simulink model "SeyyedAliSadat_DSTATCOM_FACTS_COURSE"  (R2022b)
settings: Solver=FixedStepDiscrete  StartTime=0.0  StopTime=3  FixedStep=Ts  RelTol=1e-3
InitFcn:
  |  Ts=5e-6;
undefined symbols (not defined in the file): D11, Delta, DiscIntNeverNeededParam
libraries: spsSeriesRLCBranchLib x9, spsGroundLib x6, spsThreePhaseVIMeasurementLib x4, spsSecondOrderFilterLib x4, slpidlib x4, spsLinearTransformerLib x3, spsVoltageMeasurementLib x3, spsThreePhaseParallelRLCLoadLib x2, spsUniversalBridgeLib x2, spsabctodq0Lib x2, spsPLL3phLib x2, spsPWMGenerator2LevelLib x2
(part 1 of 2)
Description:
  | Copyright 2008-2014 The MathWorks, Inc.
settings Model: Creator=MathWorks  LastModifiedBy=ali
settings SolverCC: AlgebraicLoopSolver=TrustRegion
settings DataIOCC: SaveFinalState=on  SaveFormat=Structure  SignalLoggingSaveFormat=ModelDataLogs  SaveOutput=off  SaveTime=off  ReturnWorkspaceOutputs=off  SignalLoggingName=sigsOut
settings OptimizationCC: BlockReduction=off  BooleanDataType=off  ExpressionDepthLimit=2147483647  InitFltsAndDblsToZero=on  LifeSpan=inf
settings DebuggingCC: SaveWithParameterizedLinksMsg=none  UnderspecifiedInitializationDetection=Classic  MergeDetectMultiDrivingBlocksExec=none  SignalResolutionControl=TryResolveAllWithWarning  MultiTaskDSMMsg=warning  MultiTaskCondExecSysMsg=none  FcnCallInpInsideContextMsg=warning  UnconnectedInputMsg=warning  UnconnectedOutputMsg=warning  UnconnectedLineMsg=warning  StateNameClashWarn=warning  SFUnexpectedBacktrackingDiag=warning  SFNoUnconditionalDefaultTransitionDiag=warning  SFExecutionAtInitializationDiag=none  SFMachineParentedDataDiag=warning  ArithmeticOperatorsInVariantConditions=warning
settings HardwareCC: ProdBitPerPointer=32  ProdBitPerSizeT=32  ProdBitPerPtrDiffT=32  ProdLargestAtomicFloat=None  ProdIntDivRoundTo=Undefined  ProdEndianess=Unspecified  ProdWordSize=32  ProdHWDeviceType=32-bit Generic  TargetUnknown=on
settings ModelReferenceCC: PropagateSignalLabelsOutOfModel=off
settings SFSimCC: SimUseLocalCustomCode=off  CustomCodeUndefinedFunction=UseInterfaceOnly
settings RTWCC: RTWUseLocalCustomCode=off
settings CodeAppCC: StateflowObjectComments=on
settings GRTTargetCC: TargetFcnLib=ansi_tfl_tmw.mat  TargetLangStandard=C89/C90 (ANSI)  CombineOutputUpdateFcns=off  GRTInterface=on
settings ConfigComp: CovMetricSettings=dw  CovSaveCumulativeToWorkspaceVar=on  CovSaveSingleToWorkspaceVar=on  CovExternalEMLEnable=off  CovSFcnEnable=off
settings SimscapeCC: SimscapeNormalizeSystem=off

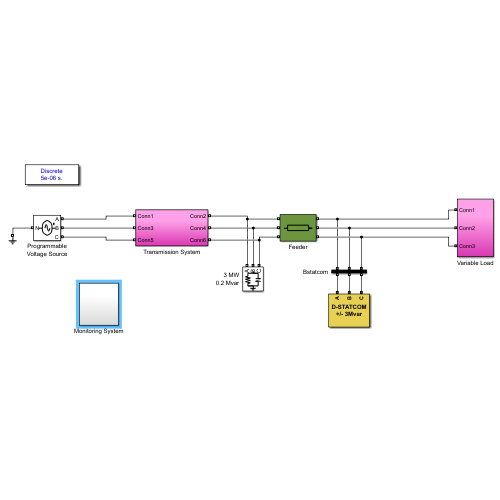
[thumbnail: Simulink's stored preview of the top-level diagram]
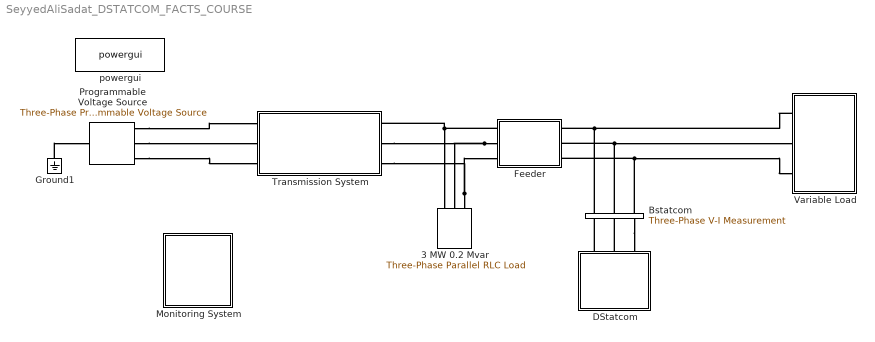
== system SeyyedAliSadat_DSTATCOM_FACTS_COURSE ==
  3 MW 0.2 Mvar : spsThreePhaseParallelRLCLoadLib/Three-Phase Parallel RLC Load  LConnTagsString=A|B|C  Configuration=Y (grounded)  NominalVoltage=33e3  Vabc=[1e3 1e3 1e3]  Vabcp=[1e3 1e3 1e3]  NominalFrequency=60  UnbalancedPower=off  ActivePower=3e6  InductivePower=0  CapacitivePower=0.2e6  Pabc=[10e3 9e3 11e3]  QLabc=[100 90 110]  QCabc=[100 90 110]  Pabcp=[10e3 9e3 11e3]  QLabcp=[100 90 110]  QCabcp=[100 90 110]  Measurements=None  LoadType=constant Z
  Bstatcom : spsThreePhaseVIMeasurementLib/Three-Phase V-I Measurement  VoltageMeasurement=phase-to-ground  SetLabelV=on  LabelV=Vabc_Bstatcom  Vpu=on  VpuLL=off  CurrentMeasurement=yes  SetLabelI=on  LabelI=Iabc_Bstatcom  Ipu=on  Pbase=3e6  Vbase=33e3  OutputType=Magnitude  PhasorSimulation=off  PSBequivalent=0
  DStatcom : Subsystem
      mask Display: disp('D-STATCOM\n+/- 3Mvar')
  Feeder : Subsystem
      mask Display: plot(0,0,100,100,[20,20,80,80,90,80,80,20,20,10],[50,40,40,50,50,50,61,61,50,50])
  Ground1 : spsGroundLib/Ground  LConnTagsString=a
  Monitoring System : Subsystem
  Programmable Voltage Source : spsThreePhaseProgrammableVoltageSourceLib/Three-Phase Programmable Voltage Source  PositiveSequence=[1.077*33e3 19 60]  VariationEntity=None  VariationType=Table of time-amplitude pairs  VariationTypeAlt=Step  VariationStep=0.5  VariationRate=10  VariationMagnitude=0.3  VariationFrequency=2  VariationTiming=[1 2]  VariationPhaseA=off  Amplitudes=[1 1.06 0.94 1.0]  TimeValues="[0 0.4  0.6   0.8 ]"  HarmonicGeneration=off  HarmonicA=[3 0.2 -25 0]  HarmonicB=[2 0.15 35 2]  Timing="[0.05  3]"  BusType=swing  Pref=0  Qref=0  Qmin=-inf  Qmax=inf
  Transmission System : Subsystem
  Variable Load : Subsystem
  powergui : spspowerguiLib/powergui  Priority=2  SimulationMode=Discrete  SampleTime=Ts  frequency=60  Iterations=50  frequencyindice=60  Pbase=100e6  ErrMax=1e-4  UnitsV=kV  UnitsW=MW  buscounter=0  FunctionMessages=off  echomessages=off  EnableUseOfTLC=off  CurrentSourceSwitches=off  DisableSnubberDevices=off  DisableRonSwitches=off  DisableVfSwitches=off  DisplayEquations=off  AutomaticDiscreteSolvers=off  SolverType=Tustin  Interpol=off  ExternalGateDelay=off  methode=off  Ts=0  x0status=blocks  SPID=off  SwTol=0  HookPort=off  NonlinearTolerance=1e-4  nMaxIteration=100  ContinueOnMaxIteration=off  RestoreLinks=warning  ResistiveCurrentMeasurement=off  Frange=[0:2:500]  Ylog=off  Xlog=on  ShowGrid=off  save=off  variable=ZData  structure=Sig1  ZoomFFT=on  StartTime=0.26  cycles=2  DisplayStyle=1  fundamental=60  FreqAxis=off  MaxFrequency=5000  frequencyindicesteady=1  RmsSteady=1  display=off
  connections:
  Bstatcom/LConn1 -- Variable Load/LConn1 -- Feeder/RConn1
  Bstatcom/LConn3 -- Feeder/RConn3 -- Variable Load/LConn3
  Ground1/LConn1 -- Programmable Voltage Source/LConn1
  Feeder/LConn1 -- Transmission System/RConn1 -- 3 MW 0.2 Mvar/LConn1
  Feeder/LConn2 -- Transmission System/RConn2 -- 3 MW 0.2 Mvar/LConn2
  Bstatcom/RConn3 -- DStatcom/RConn3
  DStatcom/RConn1 -- Bstatcom/RConn1
  DStatcom/RConn2 -- Bstatcom/RConn2
  3 MW 0.2 Mvar/LConn3 -- Feeder/LConn3 -- Transmission System/RConn3
  Programmable Voltage Source/RConn1 -- Transmission System/LConn1
  Programmable Voltage Source/RConn2 -- Transmission System/LConn2
  Programmable Voltage Source/RConn3 -- Transmission System/LConn3
  Bstatcom/LConn2 -- Feeder/RConn2 -- Variable Load/LConn2

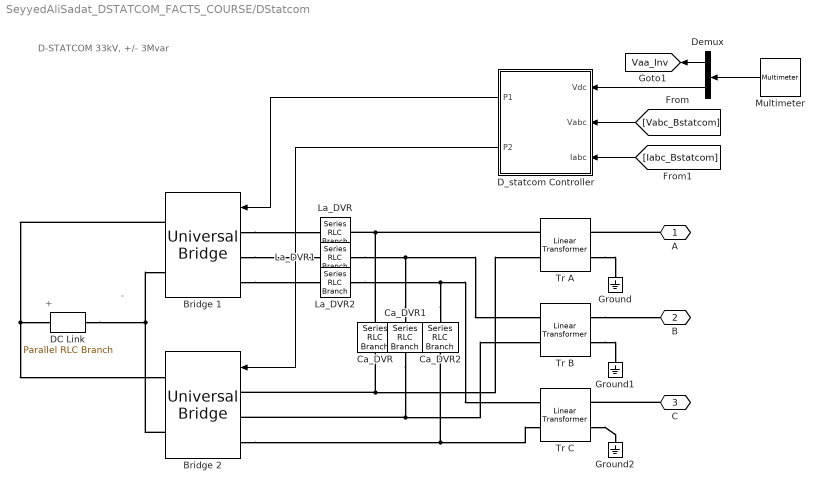
== system SeyyedAliSadat_DSTATCOM_FACTS_COURSE/DStatcom ==
  note: +
  note: -
  note: D-STATCOM
      | 33kV, +/- 3Mvar
  "Bridge 1 " : spsUniversalBridgeLib/Universal Bridge  Arms=3  SnubberResistance=1e5  SnubberCapacitance=inf  Device=IGBT / Diodes  Ron=1e-3  Lon=0  ForwardVoltages="[  2  0.8  ]"  ForwardVoltage=.8  GTOparameters=[ 10e-6 , 20e-6 ]  IGBTparameters=[ 0 0]  Measurements=Device voltages  Measurements_2=None  converterType=Rectifier
      settings: AttributesFormatString=\n
  Bridge 2 : spsUniversalBridgeLib/Universal Bridge  Arms=3  SnubberResistance=1e5  SnubberCapacitance=inf  Device=IGBT / Diodes  Ron=1e-3  Lon=0  ForwardVoltages="[  2  0.8  ]"  ForwardVoltage=.8  GTOparameters=[ 10e-6 , 20e-6 ]  IGBTparameters=[ 0 0]  Measurements=Device voltages  Measurements_2=None  converterType=Rectifier
      settings: AttributesFormatString=\n
  Ca_DVR : spsSeriesRLCBranchLib/Series RLC Branch  LConnTagsString=__new0  RConnTagsString=__new0  BranchType=RC  Resistance=100e-6*(2*pi*60)/40  Inductance=1.0  SetiL0=off  InitialCurrent=0  Capacitance=100e-6  Setx0=off  InitialVoltage=0  Measurements=None
  Ca_DVR1 : spsSeriesRLCBranchLib/Series RLC Branch  LConnTagsString=__new0  RConnTagsString=__new0  BranchType=RC  Resistance=100e-6*(2*pi*60)/40  Inductance=1.0  SetiL0=off  InitialCurrent=0  Capacitance=100e-6  Setx0=off  InitialVoltage=0  Measurements=None
  Ca_DVR2 : spsSeriesRLCBranchLib/Series RLC Branch  LConnTagsString=__new0  RConnTagsString=__new0  BranchType=RC  Resistance=100e-6*(2*pi*60)/40  Inductance=1.0  SetiL0=off  InitialCurrent=0  Capacitance=100e-6  Setx0=off  InitialVoltage=0  Measurements=None
  DC Link : spsParallelRLCBranchLib/Parallel RLC Branch  LConnTagsString=a  RConnTagsString=__new0  BranchType=C  Resistance=1.0  Inductance=1.0  SetiL0=off  InitialCurrent=0  Capacitance=5000e-6  Setx0=off  InitialVoltage=0  Measurements=Branch voltage
  D_statcom Controller : Subsystem  mask(D-STATCOM Controller){ModeOper=Voltage regulation, Vac_Ref=1.0, Qref=0, Vdc_Ref=2400, Par_VacReg=[0.55 2500], Par_VdcReg=[0.001 0.15], Par_IReg=[0.8 200 0], Ts=Ts}
      mask prompts: ModeOper "Mode of operation:"; Vac_Ref "AC voltage setpoint Vref (pu):"; Qref "Manual mode: Qref (Reactive power in pu):"; Vdc_Ref "DC Voltage setpoint (Volts)"; Par_VacReg "Vac Regulator Gains: [ Kp  Ki ]"; Par_VdcReg "Vdc Regulator Gains: [ Kp  Ki ]"; Par_IReg "Current Regulators Gain: [ Kp Ki Kd ]"; Ts "Sample time (s)"
      mask init:
      | Kp_I=Par_IReg(1);
      | Ki_I=Par_IReg(2);
      | Kd_I=Par_IReg(3);
      | Kp_Vdc=Par_VdcReg(1);
      | Ki_Vdc=Par_VdcReg(2);
      | Kp_Vac=Par_VacReg(1);
      | Ki_Vac=Par_VacReg(2);
      mask TypeOptions ModeOper: Voltage regulation | Q regulation
  Demux : Demux  Outputs=[2 1 ]
      settings: DisplayOption=none
  Ground : spsGroundLib/Ground  LConnTagsString=a
  Ground1 : spsGroundLib/Ground  LConnTagsString=a
  Ground2 : spsGroundLib/Ground  LConnTagsString=a
  La_DVR : spsSeriesRLCBranchLib/Series RLC Branch  LConnTagsString=__new0  RConnTagsString=__new0  BranchType=L  Resistance=1.0  Inductance=800e-6  SetiL0=off  InitialCurrent=0  Capacitance=1.0  Setx0=off  InitialVoltage=0  Measurements=None
  La_DVR1 : spsSeriesRLCBranchLib/Series RLC Branch  LConnTagsString=__new0  RConnTagsString=__new0  BranchType=L  Resistance=1.0  Inductance=800e-6  SetiL0=off  InitialCurrent=0  Capacitance=1.0  Setx0=off  InitialVoltage=0  Measurements=None
  La_DVR2 : spsSeriesRLCBranchLib/Series RLC Branch  LConnTagsString=__new0  RConnTagsString=__new0  BranchType=L  Resistance=1.0  Inductance=800e-6  SetiL0=off  InitialCurrent=0  Capacitance=1.0  Setx0=off  InitialVoltage=0  Measurements=None
  Multimeter : spsMultimeterLib/Multimeter  Tag=PoWeRsYsTeMmEaSuReMeNt  L=13  sel=[3 9 1]  yselected={}  Gain=[1 1 1]  OutputType=Magnitude  PlotAtSimulationStop=off  PhasorSimulation=off
      settings: AttributesFormatString=\n
  Tr A : spsLinearTransformerLib/Linear Transformer  UNITS=pu  NominalPower=[3e6/3 60]  winding1=[1250 0.03/30 0.03]  winding2=[33e3/sqrt(3) 0.03/30 0.03]  ThreeWindings=off  winding3=[60e3 0.005 0.02]  RmLm=[200 200]  Measurements=None  DataType=off
  Tr B : spsLinearTransformerLib/Linear Transformer  UNITS=pu  NominalPower=[3e6/3 60]  winding1=[1250 0.03/30 0.03]  winding2=[33e3/sqrt(3) 0.03/30 0.03]  ThreeWindings=off  winding3=[60e3 0.005 0.02]  RmLm=[200 200]  Measurements=None  DataType=off
  Tr C : spsLinearTransformerLib/Linear Transformer  UNITS=pu  NominalPower=[3e6/3 60]  winding1=[1250 0.03/30 0.03]  winding2=[33e3/sqrt(3) 0.03/30 0.03]  ThreeWindings=off  winding3=[60e3 0.005 0.02]  RmLm=[200 200]  Measurements=None  DataType=off
  A : PMIOPort  Side=Right
  B : PMIOPort  Port=2  Side=Right
  C : PMIOPort  Port=3  Side=Right
  tag scope: Vaa_Inv=global
  wires:
  Multimeter/1 -> Demux/1
  Demux/2 -> D_statcom Controller/1(Vdc)
  Demux/1 -> [Vaa_Inv]
  [Vabc_Bstatcom] -> D_statcom Controller/2(Vabc)
  [Iabc_Bstatcom] -> D_statcom Controller/3(Iabc)
  D_statcom Controller/1(P1) -> "Bridge 1 "/1
  D_statcom Controller/2(P2) -> Bridge 2/1
  connections:
  "Bridge 1 "/LConn1 -- La_DVR/LConn1
  "Bridge 1 "/LConn2 -- La_DVR1/LConn1
  "Bridge 1 "/LConn3 -- La_DVR2/LConn1
  Bridge 2/LConn2 -- Tr B/LConn2 -- Ca_DVR1/LConn1
  Bridge 2/LConn3 -- Tr C/LConn2 -- Ca_DVR2/LConn1
  Ca_DVR1/RConn1 -- La_DVR1/RConn1 -- Tr B/LConn1
  Ca_DVR2/RConn1 -- La_DVR2/RConn1 -- Tr C/LConn1
  Tr A/LConn1 -- La_DVR/RConn1 -- Ca_DVR/RConn1
  Tr C/RConn2 -- Ground2/LConn1
  Tr B/RConn2 -- Ground1/LConn1
  Tr A/RConn2 -- Ground/LConn1
  A/RConn1 -- Tr A/RConn1
  Tr B/RConn1 -- B/RConn1
  C/RConn1 -- Tr C/RConn1
  "Bridge 1 "/RConn1 -- Bridge 2/RConn1 -- DC Link/LConn1
  Bridge 2/RConn2 -- "Bridge 1 "/RConn2 -- DC Link/RConn1
  Bridge 2/LConn1 -- Tr A/LConn2 -- Ca_DVR/LConn1

== system SeyyedAliSadat_DSTATCOM_FACTS_COURSE/Feeder ==
  Three-Phase Mutual Inductance Z1-Z0 : spsThreePhaseMutualInductanceZ1Z0Lib/Three-Phase Mutual Inductance Z1-Z0  LConnTagsString=a|b|c  RConnTagsString=A|B|C  PositiveSequence="[0.1153  1.048e-3]*2"  ZeroSequence="[0.3963  2.730e-3]*2"
      settings: AttributesFormatString=\n
      settings: LibrarySourceBlock=|
      | sps_lib/Power Grid Elements/Three-Phase
      | Mutual Inductance
      | Z1-Z0
  A : PMIOPort  Side=Left
  B : PMIOPort  Port=2  Side=Left
  "C " : PMIOPort  Port=3  Side=Left
  a : PMIOPort  Port=4  Side=Right
  b : PMIOPort  Port=5  Side=Right
  c : PMIOPort  Port=6  Side=Right
  connections:
  Three-Phase Mutual Inductance Z1-Z0/RConn3 -- c/RConn1
  Three-Phase Mutual Inductance Z1-Z0/RConn2 -- b/RConn1
  Three-Phase Mutual Inductance Z1-Z0/RConn1 -- a/RConn1
  "C "/RConn1 -- Three-Phase Mutual Inductance Z1-Z0/LConn3
  B/RConn1 -- Three-Phase Mutual Inductance Z1-Z0/LConn2
  A/RConn1 -- Three-Phase Mutual Inductance Z1-Z0/LConn1

== system SeyyedAliSadat_DSTATCOM_FACTS_COURSE/Monitoring System ==
  Data Acquisition : Subsystem
  Demux : Demux  Outputs=2
  Scope1 : Scope  NumInputPorts=2
  Scope2 : Scope  NumInputPorts=4
  Scope3 : Scope  NumInputPorts=3
  Scope4 : Scope  NumInputPorts=2
  Selector : Selector  InputPortWidth=2  IndexOptions=Index vector (dialog)  Indices=2  OutputSizes=1
  wires:
  Data Acquisition/3(Iq_Iqref) -> Scope2/1  "Iq,Iqref (pu)"
  Data Acquisition/2(Va_Inv) -> Scope1/2  "Va Inv (V)"
  Data Acquisition/5(Vdc) -> Scope2/3  "Vdc (V)"
  Data Acquisition/1(VaIa) -> Selector/1, Scope1/1  "Va,Ia (pu)"
  Data Acquisition/4(PQ) -> Scope2/2  "P,Q (MVA)"
  Data Acquisition/6(m) -> Scope2/4
  Selector/1 -> Scope3/3  "Ia STAT (pu)"
  Data Acquisition/7(PQ_B3) -> Scope3/1  "PQ_B3 (MW Mvar)"
  Data Acquisition/8(VmagB1B3) -> Demux/1, Scope3/2  "V_B1 V_B3 (pu)"
  Demux/1 -> Scope4/1
  Demux/2 -> Scope4/2

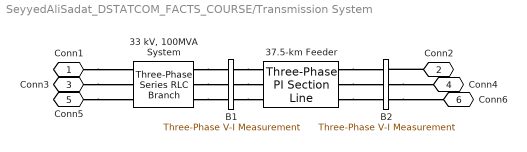
== system SeyyedAliSadat_DSTATCOM_FACTS_COURSE/Transmission System ==
  "33 kV, 100MVA System" : spsThreePhaseSeriesRLCBranchLib/Three-Phase Series RLC Branch  LConnTagsString=A|B|C  RConnTagsString=A|B|C  BranchType=RL  Resistance=33e3^2/100e6/10  Inductance=33e3^2/100e6/(2*pi*60)  Capacitance=1.0  Measurements=None
  37.5-km Feeder : spsThreePhasePISectionLineLib/Three-Phase PI Section Line  LConnTagsString=a|b|c  RConnTagsString=A|B|C  Length=37.5  Frequency=60  Resistances=[0.1153 0.3963]  Inductances=[1.048e-3 2.730e-3]  Capacitances=[11.33e-9 5.338e-9]
  B1 : spsThreePhaseVIMeasurementLib/Three-Phase V-I Measurement  VoltageMeasurement=phase-to-ground  SetLabelV=on  LabelV=Vabc_B1  Vpu=on  VpuLL=off  CurrentMeasurement=no  SetLabelI=off  LabelI=A1  Ipu=off  Pbase=100e6  Vbase=33e3  OutputType=Magnitude  PhasorSimulation=off  PSBequivalent=0
  B2 : spsThreePhaseVIMeasurementLib/Three-Phase V-I Measurement  VoltageMeasurement=phase-to-ground  SetLabelV=on  LabelV=Vabc_B2  Vpu=on  VpuLL=off  CurrentMeasurement=no  SetLabelI=off  LabelI=Iabc_B2  Ipu=off  Pbase=3e6  Vbase=33e3  OutputType=Magnitude  PhasorSimulation=off  PSBequivalent=0
  Conn1 : PMIOPort  Side=Left
  Conn2 : PMIOPort  Port=2  Side=Right
  Conn3 : PMIOPort  Port=3  Side=Left
  Conn4 : PMIOPort  Port=4  Side=Right
  Conn5 : PMIOPort  Port=5  Side=Left
  Conn6 : PMIOPort  Port=6  Side=Right
  connections:
  B1/RConn2 -- 37.5-km Feeder/LConn2
  B2/RConn3 -- Conn6/RConn1
  Conn1/RConn1 -- "33 kV, 100MVA System"/LConn1
  "33 kV, 100MVA System"/RConn3 -- B1/LConn3
  B1/RConn1 -- 37.5-km Feeder/LConn1
  B1/RConn3 -- 37.5-km Feeder/LConn3
  "33 kV, 100MVA System"/RConn2 -- B1/LConn2
  Conn5/RConn1 -- "33 kV, 100MVA System"/LConn3
  37.5-km Feeder/RConn3 -- B2/LConn3
  "33 kV, 100MVA System"/RConn1 -- B1/LConn1
  Conn3/RConn1 -- "33 kV, 100MVA System"/LConn2
  37.5-km Feeder/RConn1 -- B2/LConn1
  37.5-km Feeder/RConn2 -- B2/LConn2
  B2/RConn2 -- Conn4/RConn1
  Conn2/RConn1 -- B2/RConn1

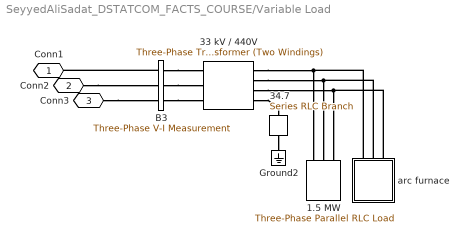
== system SeyyedAliSadat_DSTATCOM_FACTS_COURSE/Variable Load ==
  1.5 MW : spsThreePhaseParallelRLCLoadLib/Three-Phase Parallel RLC Load  LConnTagsString=A|B|C  Configuration=Y (floating)  NominalVoltage=440  Vabc=[1e3 1e3 1e3]  Vabcp=[1e3 1e3 1e3]  NominalFrequency=60  UnbalancedPower=off  ActivePower=1.5e6  InductivePower=0  CapacitivePower=0  Pabc=[10e3 9e3 11e3]  QLabc=[100 90 110]  QCabc=[100 90 110]  Pabcp=[10e3 9e3 11e3]  QLabcp=[100 90 110]  QCabcp=[100 90 110]  Measurements=None  LoadType=constant Z
  33 kV / 440V : spsThreePhaseTransformerTwoWindingsLib/Three-Phase Transformer (Two Windings)  Winding1Connection=Delta (D11)  Winding2Connection=Yn  CoreType=Three single-phase transformers  SetSaturation=off  Hysteresis=off  DataFile='basic_model'  SetInitialFlux=off  Measurements=None  UNITS=pu  NominalPower=[6e6 60]  Winding1=[33e3 , 0.05/30/2 , 0.05]  Winding2=[440 , 0.05/30/2 , 0]  Rm=500  Lm=500  L0=0.5  Saturation="[ 0,0  ;  0.005,1.2  ;  1.0,1.4 ]"  InitialFluxes=[ 0.8 , -0.8 , 0.7 ]  BreakLoop=off  DiscreteSolver=Trapezoidal iterative  DataType=off  TransfoNumber=1
  34.7 : spsSeriesRLCBranchLib/Series RLC Branch  LConnTagsString=__new0  RConnTagsString=__new0  BranchType=R  Resistance=34.7  Inductance=1.0  SetiL0=off  InitialCurrent=0  Capacitance=1.0  Setx0=off  InitialVoltage=0  Measurements=None
  B3 : spsThreePhaseVIMeasurementLib/Three-Phase V-I Measurement  VoltageMeasurement=phase-to-ground  SetLabelV=on  LabelV=Vabc_B3  Vpu=on  VpuLL=off  CurrentMeasurement=yes  SetLabelI=on  LabelI=Iabc_B3  Ipu=on  Pbase=1e6  Vbase=33e3  OutputType=Magnitude  PhasorSimulation=off  PSBequivalent=0
  Ground2 : spsGroundLib/Ground  LConnTagsString=a
  arc furnace : Subsystem  mask(Variable Load (Constant Current)){Par_Nom=[4043.48 0.85], Par_Mod=[3043.48  5], Par_Time=[0.15 1]*1, Vbase=440, Ts=Ts}
      mask prompts: Par_Nom "Nominal load: [ Current (Arms)    Power factor (0 a 1) ]"; Par_Mod "Modulation: [ Amplitude (Arms)   Frequency (Hz) ]"; Par_Time "Modulation timing : [ Ton  Toff ]"; Vbase "Nominal voltage (Volts rms ph-ph)"; Ts "Sample time:"
      mask init:
      | NomAmp=Par_Nom(1)*sqrt(2);
      | NomPha=-acos(Par_Nom(2));
      | ModFreq=Par_Mod(2);
      | ModAmp=Par_Mod(1)*sqrt(2);
      | Ton=Par_Time(1);
      | Toff=Par_Time(2);
  Conn1 : PMIOPort  Side=Left
  Conn2 : PMIOPort  Port=2  Side=Left
  Conn3 : PMIOPort  Port=3  Side=Left
  connections:
  Conn2/RConn1 -- B3/LConn2
  34.7/RConn1 -- Ground2/LConn1
  33 kV / 440V/RConn4 -- 34.7/LConn1
  B3/RConn1 -- 33 kV / 440V/LConn1
  33 kV / 440V/RConn2 -- arc furnace/LConn2 -- 1.5 MW/LConn2
  33 kV / 440V/RConn3 -- arc furnace/LConn3 -- 1.5 MW/LConn3
  B3/RConn2 -- 33 kV / 440V/LConn2
  B3/RConn3 -- 33 kV / 440V/LConn3
  33 kV / 440V/RConn1 -- arc furnace/LConn1 -- 1.5 MW/LConn1
  B3/LConn1 -- Conn1/RConn1
  Conn3/RConn1 -- B3/LConn3

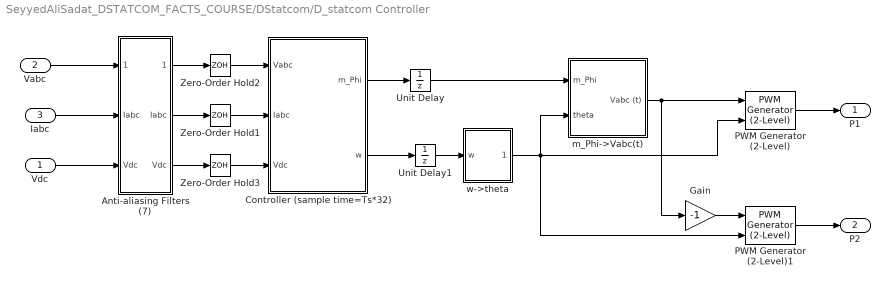
== system SeyyedAliSadat_DSTATCOM_FACTS_COURSE/DStatcom/D_statcom Controller ==
  Vdc : Inport  PortDimensions=1
  Vabc : Inport  Port=2  PortDimensions=3
  Iabc : Inport  Port=3  PortDimensions=3
  Anti-aliasing Filters (7) : Subsystem  mask(Anti-aliasing (2nd order lowpass)){Fc=2000, Ts=Ts}
      mask prompts: Fc "Cut-off frequency (Hz):"; Ts "Sample time:"
  Controller (sample time=Ts*32) : Subsystem
  Gain : Gain  Gain=-1
  PWM Generator (2-Level) : spsPWMGenerator2LevelLib/PWM Generator (2-Level)  ModulatorType=Three-phase bridge (6 pulses)  ModulatorMode=Synchronized  Fc=27*60  Pc=90  nF=28  MinMax="[ -1  1 ]"  SamplingTechnique=Natural  ModulatingSignals=off  m=0.8  Freq=60  Phase=0  Ts=Ts  ShowCarrierOutport=off
  PWM Generator (2-Level)1 : spsPWMGenerator2LevelLib/PWM Generator (2-Level)  ModulatorType=Three-phase bridge (6 pulses)  ModulatorMode=Synchronized  Fc=27*60  Pc=90  nF=28  MinMax="[ -1  1 ]"  SamplingTechnique=Natural  ModulatingSignals=off  m=0.8  Freq=60  Phase=0  Ts=Ts  ShowCarrierOutport=off
  Unit Delay : UnitDelay  SampleTime=Ts*32  HasFrameUpgradeWarning=on
  Unit Delay1 : UnitDelay  SampleTime=Ts*32  HasFrameUpgradeWarning=on
  Zero-Order Hold1 : ZeroOrderHold  SampleTime=Ts*32
  Zero-Order Hold2 : ZeroOrderHold  SampleTime=Ts*32
  Zero-Order Hold3 : ZeroOrderHold  SampleTime=Ts*32
  m_Phi->Vabc(t) : Subsystem
  w->theta : Subsystem
  P1 : Outport
  P2 : Outport  Port=2
  wires:
  Gain/1 -> PWM Generator (2-Level)1/1
  PWM Generator (2-Level)1/1 -> P2/1
  PWM Generator (2-Level)/1 -> P1/1
  Anti-aliasing Filters (7)/1(" Vabc") -> Zero-Order Hold2/1
  Anti-aliasing Filters (7)/2(Iabc) -> Zero-Order Hold1/1
  Anti-aliasing Filters (7)/3(" Vdc") -> Zero-Order Hold3/1
  Vabc/1 -> Anti-aliasing Filters (7)/1(Vabc)
  Iabc/1 -> Anti-aliasing Filters (7)/2("Iabc ")
  Vdc/1 -> Anti-aliasing Filters (7)/3("Vdc ")
  Zero-Order Hold2/1 -> Controller (sample time=Ts*32)/1(Vabc)
  Zero-Order Hold1/1 -> Controller (sample time=Ts*32)/2(Iabc)
  Zero-Order Hold3/1 -> Controller (sample time=Ts*32)/3(Vdc)
  Controller (sample time=Ts*32)/1(m_Phi) -> Unit Delay/1
  Unit Delay/1 -> m_Phi->Vabc(t)/1(m_Phi)
  Controller (sample time=Ts*32)/2(w) -> Unit Delay1/1
  Unit Delay1/1 -> w->theta/1(w)
  m_Phi->Vabc(t)/1(Vabc (t)) -> PWM Generator (2-Level)/1, Gain/1
  w->theta/1(theta) -> PWM Generator (2-Level)/2, m_Phi->Vabc(t)/2(theta), PWM Generator (2-Level)1/2

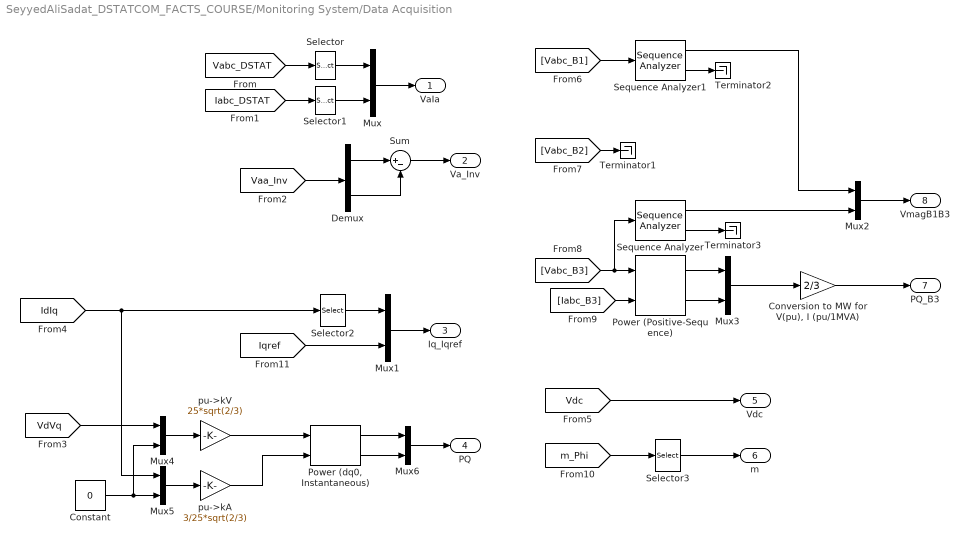
== system SeyyedAliSadat_DSTATCOM_FACTS_COURSE/Monitoring System/Data Acquisition ==
  Constant : Constant  Value=0
  "Conversion to MW for V(pu), I (pu/1MVA)" : Gain  Gain=2/3  SaturateOnIntegerOverflow=on  OutDataTypeStr=Inherit: Same as input  ParamDataTypeStr=Inherit: Same as input
  Demux : Demux  Outputs=2
      settings: DisplayOption=none
  Mux{,1..3,6} (5 alike) : Mux  Inputs=2
  Mux4 : Mux  Inputs=[2,1]
  Mux5 : Mux  Inputs=[2,1]
  Power (Positive-Sequence) : spsPowerPositiveSequenceLib/Power (Positive-Sequence)  Freq=60  Vinit=[1, 0]  Iinit=[0, 0]  Ts=Ts
      settings: LibrarySourceBlock=|
      | sps_lib/Sensors and Measurements/Power
      | (Positive-Sequence)
  "Power (dq0, Instantaneous)" : spsPowerdq0InstantaneousLib/Power (dq0, Instantaneous)
      settings: LibrarySourceBlock=|
      | sps_lib/Sensors and Measurements/Power
      | (dq0, Instantaneous)
  Selector : Selector  InputPortWidth=3  IndexOptions=Index vector (dialog)  Indices=1  OutputSizes=1
  Selector1 : Selector  InputPortWidth=3  IndexOptions=Index vector (dialog)  Indices=1  OutputSizes=1
  Selector2 : Selector  InputPortWidth=2  IndexOptions=Index vector (dialog)  Indices=2  OutputSizes=1
  Selector3 : Selector  InputPortWidth=2  IndexOptions=Index vector (dialog)  Indices=1  OutputSizes=1
  Sequence Analyzer : spsSequenceAnalyzerLib/Sequence Analyzer  Freq=60  n=1  seq=Positive  InInit=[1, 0]  Ts=Ts
      settings: LibrarySourceBlock=sps_lib/Sensors and Measurements/Sequence Analyzer
  Sequence Analyzer1 : spsSequenceAnalyzerLib/Sequence Analyzer  Freq=60  n=1  seq=Positive  InInit=[1, 0]  Ts=Ts
      settings: LibrarySourceBlock=sps_lib/Sensors and Measurements/Sequence Analyzer
  Sum : Sum  Inputs=|+-  SaturateOnIntegerOverflow=on
  Terminator1 : Terminator
  Terminator2 : Terminator
  Terminator3 : Terminator
  pu->kA : Gain  Gain=3/25*sqrt(2/3)  SaturateOnIntegerOverflow=on  OutDataTypeStr=Inherit: Same as input  ParamDataTypeStr=Inherit: Same as input
  pu->kV : Gain  Gain=25*sqrt(2/3)  SaturateOnIntegerOverflow=on  OutDataTypeStr=Inherit: Same as input  ParamDataTypeStr=Inherit: Same as input
  VaIa : Outport
  Va_Inv : Outport  Port=2
  Iq_Iqref : Outport  Port=3
  PQ : Outport  Port=4
  Vdc : Outport  Port=5
  m : Outport  Port=6
  PQ_B3 : Outport  Port=7
  VmagB1B3 : Outport  Port=8
  wires:
  [Vdc] -> Vdc/1
  Selector/1 -> Mux/1
  Selector1/1 -> Mux/2
  Mux/1 -> VaIa/1
  [m_Phi] -> Selector3/1
  [Vabc_DSTAT] -> Selector/1
  [Iabc_DSTAT] -> Selector1/1
  Mux1/1 -> Iq_Iqref/1
  Selector2/1 -> Mux1/1
  [Iqref] -> Mux1/2
  Selector3/1 -> m/1
  [Vaa_Inv] -> Demux/1
  Demux/1 -> Sum/1
  Demux/2 -> Sum/2
  Sum/1 -> Va_Inv/1
  [Vabc_B2] -> Terminator1/1
  [Vabc_B1] -> Sequence Analyzer1/1
  Mux2/1 -> VmagB1B3/1
  "Conversion to MW for V(pu), I (pu/1MVA)"/1 -> PQ_B3/1
  [Iabc_B3] -> Power (Positive-Sequence)/2
  [Vabc_B3] -> Sequence Analyzer/1, Power (Positive-Sequence)/1
  Sequence Analyzer/1 -> Mux2/2
  Power (Positive-Sequence)/1 -> Mux3/1
  Power (Positive-Sequence)/2 -> Mux3/2
  Mux3/1 -> "Conversion to MW for V(pu), I (pu/1MVA)"/1
  Sequence Analyzer/2 -> Terminator3/1
  Sequence Analyzer1/1 -> Mux2/1
  Sequence Analyzer1/2 -> Terminator2/1
  pu->kV/1 -> "Power (dq0, Instantaneous)"/1
  pu->kA/1 -> "Power (dq0, Instantaneous)"/2
  [IdIq] -> Mux5/1, Selector2/1
  [VdVq] -> Mux4/1
  Mux4/1 -> pu->kV/1
  Mux5/1 -> pu->kA/1
  "Power (dq0, Instantaneous)"/1 -> Mux6/1
  "Power (dq0, Instantaneous)"/2 -> Mux6/2
  Mux6/1 -> PQ/1
  Constant/1 -> Mux4/2, Mux5/2

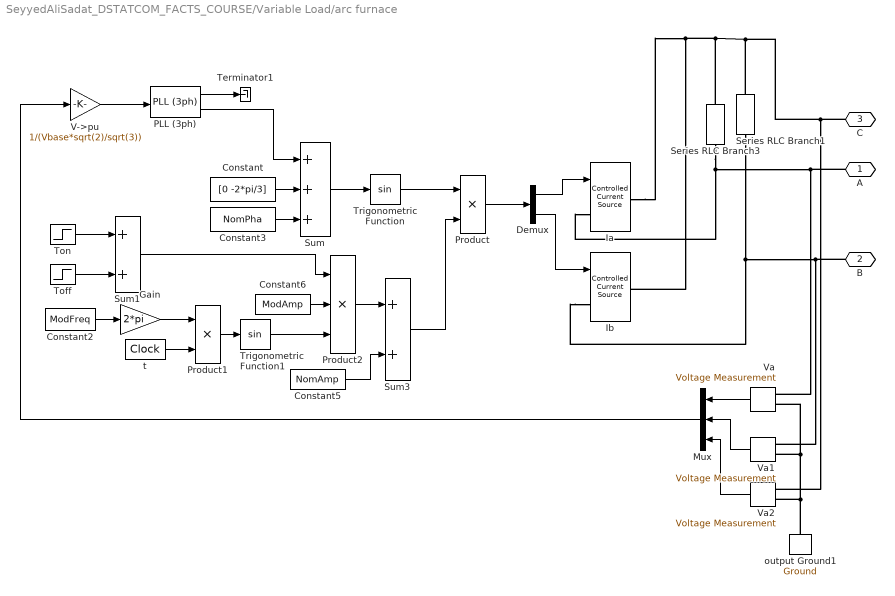
== system SeyyedAliSadat_DSTATCOM_FACTS_COURSE/Variable Load/arc furnace ==
  Constant : Constant  Value=[0 -2*pi/3]
  Constant2 : Constant  Value=ModFreq
  Constant3 : Constant  Value=NomPha
  Constant5 : Constant  Value=NomAmp
  Constant6 : Constant  Value=ModAmp
  Demux : Demux  Outputs=2
      settings: DisplayOption=none
  Gain : Gain  Gain=2*pi  SaturateOnIntegerOverflow=on  OutDataTypeStr=Inherit: Same as input  ParamDataTypeStr=Inherit: Same as input
  Ia : spsControlledCurrentSourceLib/Controlled Current Source  Description=source block  Initialize=on  Source_Type=AC  Amplitude=0  Phase=0  Frequency=0  Measurements=None
      settings: AttributesFormatString=\n
  Ib : spsControlledCurrentSourceLib/Controlled Current Source  Description=source block  Initialize=on  Source_Type=AC  Amplitude=0  Phase=0  Frequency=0  Measurements=None
      settings: AttributesFormatString=\n
  Mux : Mux  Inputs=3
  PLL (3ph) : spsPLL3phLib/PLL (3ph)  Fmin=45  Par_Init=[0, 60]  ParK=[60 1400 0]  TcD=1e-4  MaxRateChangeFreq=12  FilterCutOffFreq=25  Ts=Ts  AGC=off
  Product : Product  InputSameDT=on  SaturateOnIntegerOverflow=on  OutDataTypeStr=Inherit: Same as first input
  Product1 : Product  InputSameDT=on  SaturateOnIntegerOverflow=on  OutDataTypeStr=Inherit: Same as first input
  Product2 : Product  Inputs=3  InputSameDT=on  SaturateOnIntegerOverflow=on  OutDataTypeStr=Inherit: Same as first input
  Series RLC Branch1 : spsSeriesRLCBranchLib/Series RLC Branch  LConnTagsString=__new0  RConnTagsString=__new0  BranchType=R  Resistance=1e6  Inductance=1.0  SetiL0=off  InitialCurrent=0  Capacitance=1.0  Setx0=off  InitialVoltage=0  Measurements=None
  Series RLC Branch3 : spsSeriesRLCBranchLib/Series RLC Branch  LConnTagsString=__new0  RConnTagsString=__new0  BranchType=R  Resistance=1e6  Inductance=1.0  SetiL0=off  InitialCurrent=0  Capacitance=1.0  Setx0=off  InitialVoltage=0  Measurements=None
  Sum : Sum  Inputs=+++  InputSameDT=on  SaturateOnIntegerOverflow=on  OutDataTypeStr=Inherit: Same as first input
  Sum1 : Sum  InputSameDT=on  SaturateOnIntegerOverflow=on  OutDataTypeStr=Inherit: Same as first input
  Sum3 : Sum  InputSameDT=on  SaturateOnIntegerOverflow=on  OutDataTypeStr=Inherit: Same as first input
  Terminator1 : Terminator
  Toff : Step  Time=Toff  After=-1  SampleTime=Ts
  Ton : Step  Time=Ton  SampleTime=Ts
  Trigonometric Function : Trigonometry
  Trigonometric Function1 : Trigonometry
  V->pu : Gain  Gain=1/(Vbase*sqrt(2)/sqrt(3))  SaturateOnIntegerOverflow=on  OutDataTypeStr=Inherit: Same as input  ParamDataTypeStr=Inherit: Same as input
  Va : spsVoltageMeasurementLib/Voltage Measurement  Tag=PoWeRsYsTeMmEaSuReMeNt  PhasorSimulation=off  OutputType=Magnitude  PSBequivalent=0
  Va1 : spsVoltageMeasurementLib/Voltage Measurement  Tag=PoWeRsYsTeMmEaSuReMeNt  PhasorSimulation=off  OutputType=Magnitude  PSBequivalent=0
  Va2 : spsVoltageMeasurementLib/Voltage Measurement  Tag=PoWeRsYsTeMmEaSuReMeNt  PhasorSimulation=off  OutputType=Magnitude  PSBequivalent=0
  output Ground1 : spsGroundLib/Ground  LConnTagsString=a  RConnTagsString=__newr0
  t : DigitalClock  SampleTime=Ts
  A : PMIOPort  Side=Left
  B : PMIOPort  Port=2  Side=Left
  C : PMIOPort  Port=3  Side=Left
  wires:
  Sum1/1 -> Product2/1
  Toff/1 -> Sum1/2
  Ton/1 -> Sum1/1
  Constant6/1 -> Product2/2
  Trigonometric Function1/1 -> Product2/3
  Constant5/1 -> Sum3/2
  Product2/1 -> Sum3/1
  Sum3/1 -> Product/2
  Product1/1 -> Trigonometric Function1/1
  t/1 -> Product1/2
  Gain/1 -> Product1/1
  Constant2/1 -> Gain/1
  Constant3/1 -> Sum/3
  Mux/1 -> V->pu/1
  V->pu/1 -> PLL (3ph)/1
  Product/1 -> Demux/1
  Trigonometric Function/1 -> Product/1
  Sum/1 -> Trigonometric Function/1
  Constant/1 -> Sum/2
  Va2/1 -> Mux/3
  Va1/1 -> Mux/2
  Va/1 -> Mux/1
  Demux/1 -> Ia/1
  Demux/2 -> Ib/1
  PLL (3ph)/2 -> Sum/1
  PLL (3ph)/1 -> Terminator1/1
  connections:
  output Ground1/LConn1 -- Va2/LConn2 -- Va1/LConn2 -- Va/LConn2
  Ib/LConn1 -- Series RLC Branch1/LConn1 -- B/RConn1 -- Va1/LConn1
  Ia/LConn1 -- Series RLC Branch3/LConn1 -- A/RConn1 -- Va/LConn1
  Series RLC Branch1/RConn1 -- Series RLC Branch3/RConn1 -- Ia/RConn1 -- Ib/RConn1 -- C/RConn1 -- Va2/LConn1

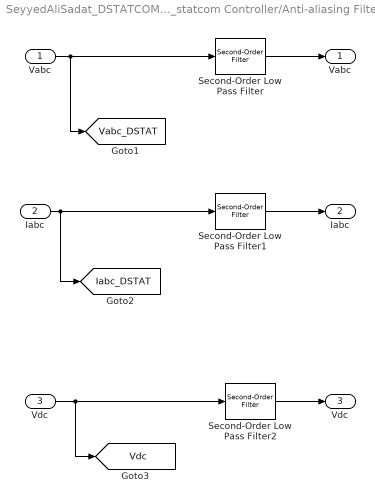
== system SeyyedAliSadat_DSTATCOM_FACTS_COURSE/DStatcom/D_statcom Controller/Anti-aliasing Filters (7) ==
  Vabc : Inport  PortDimensions=3
  "Iabc " : Inport  Port=2  PortDimensions=3
  "Vdc " : Inport  Port=3  PortDimensions=1
  Second-Order Low Pass Filter : spsSecondOrderFilterLib/Second-Order Filter  FilterType=Lowpass  Fo=Fc  Zeta=0.707  Ts=Ts  Initialize=off  Vac_Init="[0,  0,  60]"  Vdc_Init=0  PlotResponse=off  FreqRange=[0, 500, 1]
      settings: AttributesFormatString=f0: %<Fo>
      settings: LibrarySourceBlock=|
      | sps_lib/Control/Filters/Second-Order
      | Filter
  Second-Order Low Pass Filter1 : spsSecondOrderFilterLib/Second-Order Filter  FilterType=Lowpass  Fo=Fc  Zeta=0.707  Ts=Ts  Initialize=off  Vac_Init="[0,  0,  60]"  Vdc_Init=0  PlotResponse=off  FreqRange=[0, 500, 1]
      settings: AttributesFormatString=f0: %<Fo>
      settings: LibrarySourceBlock=|
      | sps_lib/Control/Filters/Second-Order
      | Filter
  Second-Order Low Pass Filter2 : spsSecondOrderFilterLib/Second-Order Filter  FilterType=Lowpass  Fo=Fc  Zeta=0.707  Ts=Ts  Initialize=off  Vac_Init="[0,  0,  60]"  Vdc_Init=0  PlotResponse=off  FreqRange=[0, 500, 1]
      settings: AttributesFormatString=f0: %<Fo>
      settings: LibrarySourceBlock=|
      | sps_lib/Control/Filters/Second-Order
      | Filter
  " Vabc" : Outport
  Iabc : Outport  Port=2
  " Vdc" : Outport  Port=3
  tag scope: Iabc_DSTAT=global, Vabc_DSTAT=global, Vdc=global
  wires:
  Second-Order Low Pass Filter/1 -> " Vabc"/1
  Second-Order Low Pass Filter1/1 -> Iabc/1
  "Iabc "/1 -> [Iabc_DSTAT], Second-Order Low Pass Filter1/1
  Vabc/1 -> [Vabc_DSTAT], Second-Order Low Pass Filter/1
  "Vdc "/1 -> [Vdc], Second-Order Low Pass Filter2/1
  Second-Order Low Pass Filter2/1 -> " Vdc"/1

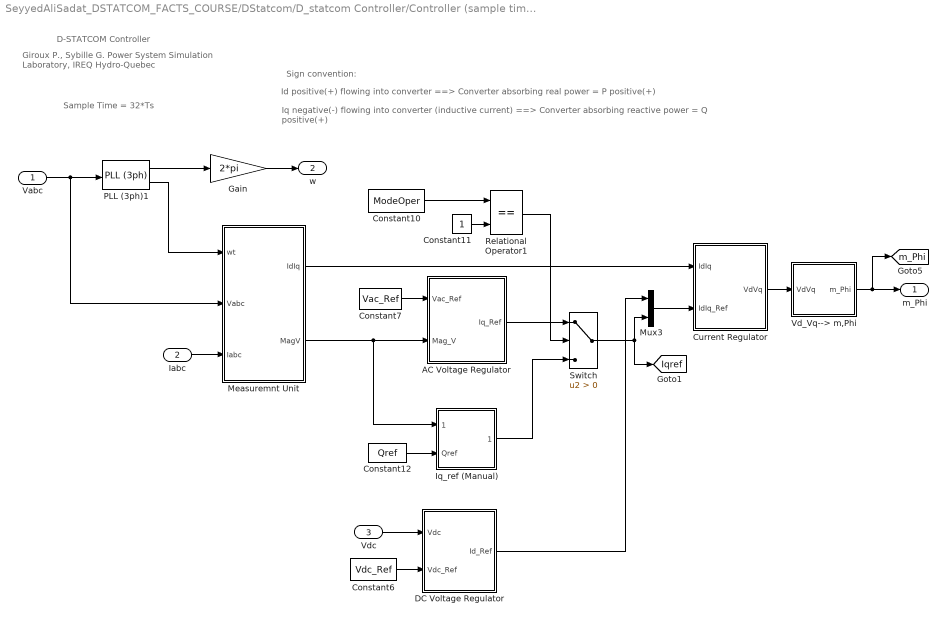
== system SeyyedAliSadat_DSTATCOM_FACTS_COURSE/DStatcom/D_statcom Controller/Controller (sample time=Ts*32) ==
  note: Sample Time = 32*Ts
  note: Id positive(+) flowing into converter ==> Converter absorbing real power = P positive(+)
  note: Sign convention:
  note: Iq negative(-) flowing into converter (inductive current) ==> Converter absorbing reactive power = Q positive(+)
  note: Giroux P., Sybille G.
      | Power System Simulation Laboratory, IREQ
      | Hydro-Quebec
  note: D-STATCOM Controller
  Vabc : Inport  PortDimensions=3
  Iabc : Inport  Port=2  PortDimensions=3
  Vdc : Inport  Port=3  PortDimensions=1
  AC Voltage Regulator : Subsystem  mask(DC Voltage regulator){Kp=Kp_Vac, Ki=Ki_Vac, Ts=32*Ts}
      mask prompts: Kp "Proportional gain (Kp):"; Ki "Integral gain(Ki)"; Ts "Sample time:"
  Constant10 : Constant  Value=ModeOper
  Constant11 : Constant
  Constant12 : Constant  Value=Qref
  Constant6 : Constant  Value=Vdc_Ref
  Constant7 : Constant  Value=Vac_Ref
  Current Regulator : Subsystem  mask(Current Regulators){Kp=Kp_I, Ki=Ki_I, Par_Limits=[1 -1], Init=0, Ts=32*Ts}
      mask prompts: Kp "Proportional gain (Kp):"; Ki "Integral gain (Ki):"; Par_Limits "Output limits: [ Upper   Lower ]"; Init "Output initial value:"; Ts "Sample time:"
      mask help:
      | Sign convention:
      | Id positive(+) flowing into converter ==> Converter absorbing real power = P positive(+)
      | Iq negative(-) flowing into converter (inductive current) ==> Converter absorbing reactive power = Q positive(+)
  DC Voltage Regulator : Subsystem  mask(DC Voltage regulator){Kp=Kp_Vdc, Ki=Ki_Vdc, Ts=32*Ts}
      mask prompts: Kp "Proportional gain (Kp):"; Ki "Integral gain(Ki)"; Ts "Sample time:"
  Gain : Gain  Gain=2*pi
  Iq_ref (Manual) : Subsystem
  Measuremnt Unit : Subsystem
  Mux3 : Mux  Inputs=2
  PLL (3ph)1 : spsPLL3phLib/PLL (3ph)  Fmin=45  Par_Init=[3.7 60]  ParK=[60 1400 0]  TcD=1.6e-4  MaxRateChangeFreq=10  FilterCutOffFreq=25  Ts=32*Ts  AGC=off
  Relational Operator1 : RelationalOperator  Operator===
  Switch : Switch  Criteria=u2 > Threshold
  Vd_Vq--> m,Phi : Subsystem
  m_Phi : Outport
  w : Outport  Port=2
  tag scope: Iqref=global, m_Phi=global
  wires:
  Gain/1 -> w/1
  PLL (3ph)1/1 -> Gain/1
  PLL (3ph)1/2 -> Measuremnt Unit/1(wt)
  Vabc/1 -> Measuremnt Unit/2(Vabc), PLL (3ph)1/1
  Constant6/1 -> DC Voltage Regulator/2(Vdc_Ref)
  Vdc/1 -> DC Voltage Regulator/1(Vdc)
  Constant11/1 -> Relational Operator1/2
  Constant10/1 -> Relational Operator1/1
  Constant12/1 -> Iq_ref (Manual)/2(Qref)
  Iabc/1 -> Measuremnt Unit/3(Iabc)
  Measuremnt Unit/2(MagV) -> AC Voltage Regulator/2(Mag_V), Iq_ref (Manual)/1(MagV)
  Constant7/1 -> AC Voltage Regulator/1(Vac_Ref)
  Measuremnt Unit/1(IdIq) -> Current Regulator/1(IdIq)
  AC Voltage Regulator/1(Iq_Ref) -> Switch/1
  Mux3/1 -> Current Regulator/2(IdIq_Ref)
  Switch/1 -> Mux3/2, [Iqref]
  DC Voltage Regulator/1(Id_Ref) -> Mux3/1
  Iq_ref (Manual)/1(Iqref*) -> Switch/3
  Relational Operator1/1 -> Switch/2
  Current Regulator/1(VdVq) -> Vd_Vq--> m,Phi/1(VdVq)
  Vd_Vq--> m,Phi/1(m_Phi) -> m_Phi/1, [m_Phi]

== system SeyyedAliSadat_DSTATCOM_FACTS_COURSE/DStatcom/D_statcom Controller/m_Phi->Vabc(t) ==
  m_Phi : Inport
  theta : Inport  Port=2
  Constant1 : Constant  Value=[0 -2*pi/3 2*pi/3]
  Demux : Demux  Outputs=2
      settings: DisplayOption=none
  Product2 : Product  InputSameDT=on  SaturateOnIntegerOverflow=on  OutDataTypeStr=Inherit: Same as first input
  Sum4 : Sum  Inputs=+++  InputSameDT=on  SaturateOnIntegerOverflow=on  OutDataTypeStr=Inherit: Same as first input
  Trigonometric Function1 : Trigonometry
  deg. ->rad : Gain  Gain=pi/180  SaturateOnIntegerOverflow=on  OutDataTypeStr=Inherit: Same as input  ParamDataTypeStr=Inherit: Same as input
  Vabc (t) : Outport
  wires:
  Trigonometric Function1/1 -> Product2/2
  Sum4/1 -> Trigonometric Function1/1
  Constant1/1 -> Sum4/2
  Demux/1 -> Product2/1
  Product2/1 -> Vabc (t)/1
  m_Phi/1 -> Demux/1
  deg. ->rad/1 -> Sum4/1
  theta/1 -> Sum4/3
  Demux/2 -> deg. ->rad/1

== system SeyyedAliSadat_DSTATCOM_FACTS_COURSE/DStatcom/D_statcom Controller/w->theta ==
  w : Inport
  Constant4 : Constant  Value=2*pi
  Discrete-Time Integrator : DiscreteIntegrator  SampleTime=Ts  ICPrevOutput=DiscIntNeverNeededParam  ICPrevScaledInput=DiscIntNeverNeededParam
  Math Function : Math  Operator=mod  SignedPower=on
  theta : Outport
  wires:
  Math Function/1 -> theta/1
  w/1 -> Discrete-Time Integrator/1
  Constant4/1 -> Math Function/2
  Discrete-Time Integrator/1 -> Math Function/1

== system SeyyedAliSadat_DSTATCOM_FACTS_COURSE/DStatcom/D_statcom Controller/Controller (sample time=Ts*32)/AC Voltage Regulator ==
  Vac_Ref : Inport
  Mag_V : Inport  Port=2
  Discrete PI Controller : slpidlib/PID Controller  Controller=PI  Form=Parallel  TimeDomain=Discrete-time  UseExternalTs=off  SampleTime=Ts  IntegratorMethod=Forward Euler  FilterMethod=Forward Euler  ControllerParametersSource=internal  P=Kp  I=Ki  UseKiTs=off  D=0  N=100  UseFilter=on  TunerSelectOption=Transfer Function Based (PID Tuner App)  InitialConditionSource=internal  InitialConditionForIntegrator=0  InitialConditionForFilter=0  DifferentiatorICPrevScaledInput=0  ExternalReset=none  TrackingMode=off  Kt=1  LimitOutput=on  SatLimitsSource=internal  UpperSaturationLimit=1  LowerSaturationLimit=-1  LinearizeAsGain=off  AntiWindupMode=clamping  Kb=1  LimitIntegrator=off  UpperIntegratorSaturationLimit=inf  LowerIntegratorSaturationLimit=-inf  POutMin=[]  POutMax=[]  IOutMin=[]  IOutMax=[]  DOutMin=[]  DOutMax=[]  NOutMin=[]  NOutMax=[]  SumOutMin=[]  SumOutMax=[]  SaturationOutMin=[]  SaturationOutMax=[]  PParamMin=[]  PParamMax=[]  IParamMin=[]  IParamMax=[]  DParamMin=[]  DParamMax=[]  NParamMin=[]  NParamMax=[]  KbParamMin=[]  KbParamMax=[]  KtParamMin=[]  KtParamMax=[]  KbOutMin=[]  KbOutMax=[]  KtOutMin=[]  KtOutMax=[]  IntegratorOutMin=[]  IntegratorOutMax=[]  FilterOutMin=[]  FilterOutMax=[]  SumI1OutMin=[]  SumI1OutMax=[]  SumI2OutMin=[]  SumI2OutMax=[]  SumI3OutMin=[]  SumI3OutMax=[]  SumI4OutMin=[]  SumI4OutMax=[]  SumDOutMin=[]  SumDOutMax=[]  DifferentiatorOutMin=[]  DifferentiatorOutMax=[]  FilterDiffOutCoefMin=[]  FilterDiffOutCoefMax=[]  ReciprocalOutMin=[]  ReciprocalOutMax=[]  SumDenOutMin=[]  SumDenOutMax=[]  SumNumOutMin=[]  SumNumOutMax=[]  DivideOutMin=[]  DivideOutMax=[]  UdiffTsProdOutMin=[]  UdiffTsProdOutMax=[]  NTsProdOutMin=[]  NTsProdOutMax=[]  UintegralTsProdOutMin=[]  UintegralTsProdOutMax=[]  UngainTsProdOutMin=[]  UngainTsProdOutMax=[]  ClampingZeroOutDataTypeStr=Inherit: Inherit via back propagation  ClampingZeroOutMin=[]  ClampingZeroOutMax=[]  FilterDenConstantOutDataTypeStr=Inherit: Inherit via back propagation  FilterDenConstantOutMin=[]  FilterDenConstantOutMax=[]  PCopyOutDataTypeStr=Inherit: Inherit via back propagation  PCopyOutMin=[]  PCopyOutMax=[]  NCopyOutDataTypeStr=Inherit: Inherit via back propagation  NCopyOutMin=[]  NCopyOutMax=[]  IntegratorContinuousStateAttributes=''  IntegratorStateMustResolveToSignalObject=off  IntegratorRTWStateStorageClass=Auto  FilterContinuousStateAttributes=''  FilterStateMustResolveToSignalObject=off  FilterRTWStateStorageClass=Auto  ParallelPVariant=InternalParameters  IdealPVariant=Disabled  IVariant=InternalParameters  DVariant=Disabled  IntegratorVariant=Discrete  SatVariant=Enabled  AWVariant=DiscClampingParallel  PCopyVariant=Disabled  TRVariant=Disabled  FdbkBlocksVariant=Forward  IdealPFdbkVariant=Disabled  SatFdbkVariant=Disabled  DerivativeFilterVariant=Disabled  NVariant=Disabled  NCopyVariant=Disabled_SignalSpec  FilterICVariant=Disabled  IntegratorICVariant=InternalICs  ExternalResetVariant=Disabled  TRSumVariant=Passthrough  SumFdbkVariant=Disabled  SumVariant=Sum_PI  TsampFilterVariant=InternalTs  TsampNgainVariant=Passthrough  TsampIntegralVariant=Passthrough  ExternalSaturationOutDataTypeStr=Inherit: Same as second input
      settings: AttributesFormatString=P = %<P>\nI = %<I>
  Sum : Sum  Inputs=|+-  InputSameDT=on  SaturateOnIntegerOverflow=on  OutDataTypeStr=Inherit: Same as first input
  Iq_Ref : Outport  InitialOutput=0
  wires:
  Discrete PI Controller/1 -> Iq_Ref/1
  Sum/1 -> Discrete PI Controller/1
  Mag_V/1 -> Sum/2
  Vac_Ref/1 -> Sum/1

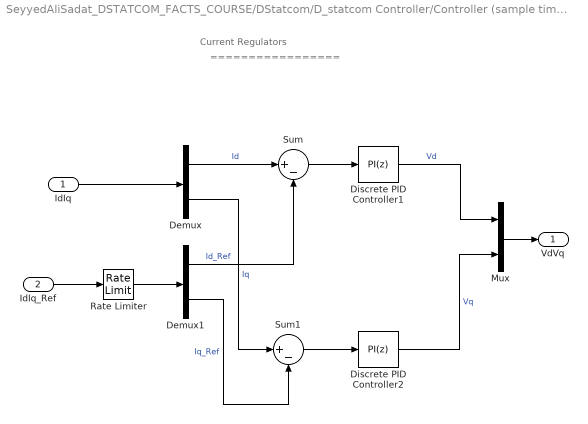
== system SeyyedAliSadat_DSTATCOM_FACTS_COURSE/DStatcom/D_statcom Controller/Controller (sample time=Ts*32)/Current Regulator ==
  note: Current Regulators
  note: =================
  IdIq : Inport  PortDimensions=2
  IdIq_Ref : Inport  Port=2  PortDimensions=2
  Demux : Demux  Outputs=2
      settings: DisplayOption=none
  Demux1 : Demux  Outputs=2
      settings: DisplayOption=none
  Discrete PID Controller1 : slpidlib/PID Controller  Controller=PI  Form=Parallel  TimeDomain=Discrete-time  UseExternalTs=off  SampleTime=Ts  IntegratorMethod=Forward Euler  FilterMethod=Forward Euler  ControllerParametersSource=internal  P=Kp  I=Ki  UseKiTs=off  D=0  N=100  UseFilter=on  TunerSelectOption=Transfer Function Based (PID Tuner App)  InitialConditionSource=internal  InitialConditionForIntegrator=0  InitialConditionForFilter=0  DifferentiatorICPrevScaledInput=0  ExternalReset=none  TrackingMode=off  Kt=1  LimitOutput=on  SatLimitsSource=internal  UpperSaturationLimit=1  LowerSaturationLimit=-1  LinearizeAsGain=off  AntiWindupMode=clamping  Kb=1  LimitIntegrator=off  UpperIntegratorSaturationLimit=inf  LowerIntegratorSaturationLimit=-inf  POutMin=[]  POutMax=[]  IOutMin=[]  IOutMax=[]  DOutMin=[]  DOutMax=[]  NOutMin=[]  NOutMax=[]  SumOutMin=[]  SumOutMax=[]  SaturationOutMin=[]  SaturationOutMax=[]  PParamMin=[]  PParamMax=[]  IParamMin=[]  IParamMax=[]  DParamMin=[]  DParamMax=[]  NParamMin=[]  NParamMax=[]  KbParamMin=[]  KbParamMax=[]  KtParamMin=[]  KtParamMax=[]  KbOutMin=[]  KbOutMax=[]  KtOutMin=[]  KtOutMax=[]  IntegratorOutMin=[]  IntegratorOutMax=[]  FilterOutMin=[]  FilterOutMax=[]  SumI1OutMin=[]  SumI1OutMax=[]  SumI2OutMin=[]  SumI2OutMax=[]  SumI3OutMin=[]  SumI3OutMax=[]  SumI4OutMin=[]  SumI4OutMax=[]  SumDOutMin=[]  SumDOutMax=[]  DifferentiatorOutMin=[]  DifferentiatorOutMax=[]  FilterDiffOutCoefMin=[]  FilterDiffOutCoefMax=[]  ReciprocalOutMin=[]  ReciprocalOutMax=[]  SumDenOutMin=[]  SumDenOutMax=[]  SumNumOutMin=[]  SumNumOutMax=[]  DivideOutMin=[]  DivideOutMax=[]  UdiffTsProdOutMin=[]  UdiffTsProdOutMax=[]  NTsProdOutMin=[]  NTsProdOutMax=[]  UintegralTsProdOutMin=[]  UintegralTsProdOutMax=[]  UngainTsProdOutMin=[]  UngainTsProdOutMax=[]  ClampingZeroOutDataTypeStr=Inherit: Inherit via back propagation  ClampingZeroOutMin=[]  ClampingZeroOutMax=[]  FilterDenConstantOutDataTypeStr=Inherit: Inherit via back propagation  FilterDenConstantOutMin=[]  FilterDenConstantOutMax=[]  PCopyOutDataTypeStr=Inherit: Inherit via back propagation  PCopyOutMin=[]  PCopyOutMax=[]  NCopyOutDataTypeStr=Inherit: Inherit via back propagation  NCopyOutMin=[]  NCopyOutMax=[]  IntegratorContinuousStateAttributes=''  IntegratorStateMustResolveToSignalObject=off  IntegratorRTWStateStorageClass=Auto  FilterContinuousStateAttributes=''  FilterStateMustResolveToSignalObject=off  FilterRTWStateStorageClass=Auto  ParallelPVariant=InternalParameters  IdealPVariant=Disabled  IVariant=InternalParameters  DVariant=Disabled  IntegratorVariant=Discrete  SatVariant=Enabled  AWVariant=DiscClampingParallel  PCopyVariant=Disabled  TRVariant=Disabled  FdbkBlocksVariant=Forward  IdealPFdbkVariant=Disabled  SatFdbkVariant=Disabled  DerivativeFilterVariant=Disabled  NVariant=Disabled  NCopyVariant=Disabled_SignalSpec  FilterICVariant=Disabled  IntegratorICVariant=InternalICs  ExternalResetVariant=Disabled  TRSumVariant=Passthrough  SumFdbkVariant=Disabled  SumVariant=Sum_PI  TsampFilterVariant=InternalTs  TsampNgainVariant=Passthrough  TsampIntegralVariant=Passthrough  ExternalSaturationOutDataTypeStr=Inherit: Same as second input
      settings: AttributesFormatString=P = %<P>\nI = %<I>
  Discrete PID Controller2 : slpidlib/PID Controller  Controller=PI  Form=Parallel  TimeDomain=Discrete-time  UseExternalTs=off  SampleTime=Ts  IntegratorMethod=Forward Euler  FilterMethod=Forward Euler  ControllerParametersSource=internal  P=Kp  I=Ki  UseKiTs=off  D=0  N=100  UseFilter=on  TunerSelectOption=Transfer Function Based (PID Tuner App)  InitialConditionSource=internal  InitialConditionForIntegrator=0  InitialConditionForFilter=0  DifferentiatorICPrevScaledInput=0  ExternalReset=none  TrackingMode=off  Kt=1  LimitOutput=on  SatLimitsSource=internal  UpperSaturationLimit=1  LowerSaturationLimit=-1  LinearizeAsGain=off  AntiWindupMode=clamping  Kb=1  LimitIntegrator=off  UpperIntegratorSaturationLimit=inf  LowerIntegratorSaturationLimit=-inf  POutMin=[]  POutMax=[]  IOutMin=[]  IOutMax=[]  DOutMin=[]  DOutMax=[]  NOutMin=[]  NOutMax=[]  SumOutMin=[]  SumOutMax=[]  SaturationOutMin=[]  SaturationOutMax=[]  PParamMin=[]  PParamMax=[]  IParamMin=[]  IParamMax=[]  DParamMin=[]  DParamMax=[]  NParamMin=[]  NParamMax=[]  KbParamMin=[]  KbParamMax=[]  KtParamMin=[]  KtParamMax=[]  KbOutMin=[]  KbOutMax=[]  KtOutMin=[]  KtOutMax=[]  IntegratorOutMin=[]  IntegratorOutMax=[]  FilterOutMin=[]  FilterOutMax=[]  SumI1OutMin=[]  SumI1OutMax=[]  SumI2OutMin=[]  SumI2OutMax=[]  SumI3OutMin=[]  SumI3OutMax=[]  SumI4OutMin=[]  SumI4OutMax=[]  SumDOutMin=[]  SumDOutMax=[]  DifferentiatorOutMin=[]  DifferentiatorOutMax=[]  FilterDiffOutCoefMin=[]  FilterDiffOutCoefMax=[]  ReciprocalOutMin=[]  ReciprocalOutMax=[]  SumDenOutMin=[]  SumDenOutMax=[]  SumNumOutMin=[]  SumNumOutMax=[]  DivideOutMin=[]  DivideOutMax=[]  UdiffTsProdOutMin=[]  UdiffTsProdOutMax=[]  NTsProdOutMin=[]  NTsProdOutMax=[]  UintegralTsProdOutMin=[]  UintegralTsProdOutMax=[]  UngainTsProdOutMin=[]  UngainTsProdOutMax=[]  ClampingZeroOutDataTypeStr=Inherit: Inherit via back propagation  ClampingZeroOutMin=[]  ClampingZeroOutMax=[]  FilterDenConstantOutDataTypeStr=Inherit: Inherit via back propagation  FilterDenConstantOutMin=[]  FilterDenConstantOutMax=[]  PCopyOutDataTypeStr=Inherit: Inherit via back propagation  PCopyOutMin=[]  PCopyOutMax=[]  NCopyOutDataTypeStr=Inherit: Inherit via back propagation  NCopyOutMin=[]  NCopyOutMax=[]  IntegratorContinuousStateAttributes=''  IntegratorStateMustResolveToSignalObject=off  IntegratorRTWStateStorageClass=Auto  FilterContinuousStateAttributes=''  FilterStateMustResolveToSignalObject=off  FilterRTWStateStorageClass=Auto  ParallelPVariant=InternalParameters  IdealPVariant=Disabled  IVariant=InternalParameters  DVariant=Disabled  IntegratorVariant=Discrete  SatVariant=Enabled  AWVariant=DiscClampingParallel  PCopyVariant=Disabled  TRVariant=Disabled  FdbkBlocksVariant=Forward  IdealPFdbkVariant=Disabled  SatFdbkVariant=Disabled  DerivativeFilterVariant=Disabled  NVariant=Disabled  NCopyVariant=Disabled_SignalSpec  FilterICVariant=Disabled  IntegratorICVariant=InternalICs  ExternalResetVariant=Disabled  TRSumVariant=Passthrough  SumFdbkVariant=Disabled  SumVariant=Sum_PI  TsampFilterVariant=InternalTs  TsampNgainVariant=Passthrough  TsampIntegralVariant=Passthrough  ExternalSaturationOutDataTypeStr=Inherit: Same as second input
      settings: AttributesFormatString=P = %<P>\nI = %<I>
  Mux : Mux  Inputs=2
  Rate Limiter : RateLimiter  RisingSlewLimit=240  FallingSlewLimit=-240  SampleTimeMode=inherited
      settings: AttributesFormatString=Up = %<RisingSlewLimit>\nDown = %<FallingSlewLimit>\nIC = %<InitialCondition>
  Sum : Sum  Inputs=|+-  InputSameDT=on  SaturateOnIntegerOverflow=on  OutDataTypeStr=Inherit: Same as first input
  Sum1 : Sum  Inputs=|+-  InputSameDT=on  SaturateOnIntegerOverflow=on  OutDataTypeStr=Inherit: Same as first input
  VdVq : Outport
  wires:
  Discrete PID Controller2/1 -> Mux/2  "Vq"
  Discrete PID Controller1/1 -> Mux/1  "Vd"
  IdIq/1 -> Demux/1
  Demux/1 -> Sum/1  "Id"
  Demux1/1 -> Sum/2  "Id_Ref"
  Demux/2 -> Sum1/1  "Iq"
  Sum1/1 -> Discrete PID Controller2/1
  Demux1/2 -> Sum1/2  "Iq_Ref"
  Sum/1 -> Discrete PID Controller1/1
  Mux/1 -> VdVq/1
  IdIq_Ref/1 -> Rate Limiter/1
  Rate Limiter/1 -> Demux1/1
